simulink model "s8_15"  (Simulink 6.6)
settings: Solver=ode23  SolverMode=SingleTasking  StartTime=0.0  StopTime=t_d  MaxStep=Tc  RelTol=1e-8  AbsTol=1e-8
values from neighbouring files (symbols this model uses):
  F_v = K_r*diag([0.01 0.01])*K_r    [i8_15.m]
  g = 9.81    [i8_15.m]
  K_d = 3250*diag([1 1])    [i8_15.m]
  K_p = 16250*diag([1 1])    [i8_15.m]
  p_d = [0.6; -0.2]    [i8_15.m]
  pi_m = pi_l    [i8_15.m]
  q_i = inv_k2u(a,p_i)    [i8_15.m]
  Tc = 0.001    [i8_15.m]
  Ts = Tc    (= 0.001)    [i8_15.m]
undefined symbols (not defined in the file or in its folder): a, iner_l, pi_l
settings Model: Creator=luigivillani  LastModifiedBy=luigivillani  ExtModeAutoUpdateStatusClock=off
settings SolverCC: InitialStep=0.1*Tc
settings DataIOCC: LimitDataPoints=off  SaveOutput=off  SaveTime=off
settings OptimizationCC: BlockReduction=off  BooleanDataType=off
settings DebuggingCC: SignalResolutionControl=TryResolveAllWithWarning  SolverPrmCheckMsg=none  MultiTaskDSMMsg=warning  MultiTaskCondExecSysMsg=none  StrictBusMsg=None
settings HardwareCC: TargetUnknown=on
settings RTWCC: IncludeERTFirstTime=on

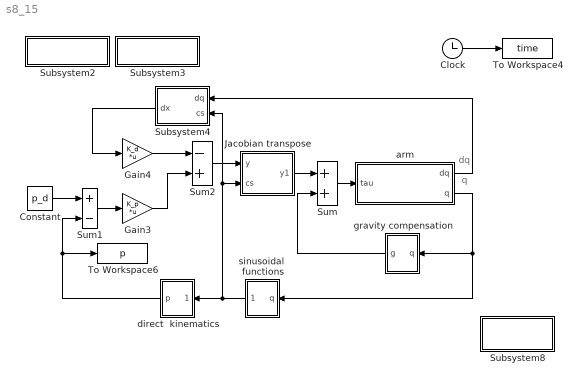
== system s8_15 ==
  note: dq
  note: q
  Clock : Clock
  Constant : Constant  Value=p_d
  Gain3 : Gain  Gain=K_p  Multiplication=Matrix(K*u)  SampleTime=Tc
      mask Display: disp('K_p')
  Gain4 : Gain  Gain=K_d  Multiplication=Matrix(K*u)  SampleTime=Tc
      mask Display: disp('K_d')
  Jacobian transpose : Subsystem
      mask Display: disp('tr(J_a(q))')
  Subsystem2 : Subsystem
      settings: OpenFcn=clear all;c=0;i8_15;
      mask Display: disp('p_d=[0.5 0.5]')
  Subsystem3 : Subsystem
      settings: OpenFcn=clear all;c=1;i8_15;
      mask Display: disp('p_d=[0.6 -0.2]')
  Subsystem4 : Subsystem  Orientation=left
      mask Display: disp('J_a(q)')
  Subsystem8 : Subsystem  Orientation=left
      settings: OpenFcn=p8_15;
      mask Display: disp('plot')
  Sum : Sum  SaturateOnIntegerOverflow=on  InputSameDT=on
  Sum1 : Sum  Inputs=+-  SaturateOnIntegerOverflow=on  InputSameDT=on
  Sum2 : Sum  Inputs=-+  SaturateOnIntegerOverflow=on  InputSameDT=on
  To Workspace4 : ToWorkspace  VariableName=time  SampleTime=Ts  SaveFormat=Array
      settings: MaxDataPoints=4001
  To Workspace6 : ToWorkspace  VariableName=p  SampleTime=Ts  SaveFormat=Array
      settings: MaxDataPoints=4001
  arm : Subsystem
      mask Display: disp('inv(B(q))(tau-tau'')')
  direct  kinematics : Subsystem  Orientation=left
      mask Display: disp('k(q)')
  gravity compensation : Subsystem  Orientation=left
      mask Display: disp('g(q)')
  sinusoidal  functions : Subsystem  Orientation=left
      mask Display: disp('cs(q)')
  wires:
  Sum/1 -> arm/1(tau)
  Sum1/1 -> Gain3/1
  Clock/1 -> To Workspace4/1
  Constant/1 -> Sum1/1
  gravity compensation/1(g) -> Sum/2
  Jacobian transpose/1(y1) -> Sum/1
  arm/2("q ") -> gravity compensation/1(q), sinusoidal  functions/1(q)
  Sum2/1 -> Jacobian transpose/1(y)
  Gain4/1 -> Sum2/1
  Subsystem4/1(dx) -> Gain4/1
  Gain3/1 -> Sum2/2
  arm/1(dq) -> Subsystem4/1(dq)
  sinusoidal  functions/1(cs) -> Subsystem4/2(cs), Jacobian transpose/2(cs), direct  kinematics/1(cs)
  direct  kinematics/1(p) -> Sum1/2, To Workspace6/1

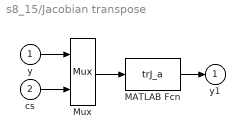
== system s8_15/Jacobian transpose ==
  y : Inport
  cs : Inport  Port=2
  MATLAB Fcn : MATLABFcn  MATLABFcn=trJ_a  OutputDimensions=2  SampleTime=Tc
      mask Display: disp('J''_a(q)y')
  Mux : Mux  Inputs=[2,4]
  y1 : Outport  InitialOutput=0
  wires:
  MATLAB Fcn/1 -> y1/1
  Mux/1 -> MATLAB Fcn/1
  cs/1 -> Mux/2
  y/1 -> Mux/1

== system s8_15/Subsystem2 ==
  note: start

== system s8_15/Subsystem3 ==
  note: start

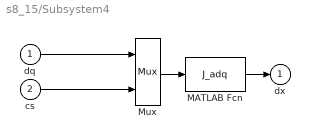
== system s8_15/Subsystem4 ==
  dq : Inport
  cs : Inport  Port=2
  MATLAB Fcn : MATLABFcn  MATLABFcn=J_adq  OutputDimensions=2  SampleTime=Tc
      mask Display: disp('J_a(q)dq')
  Mux : Mux  Inputs=[2,4]
  dx : Outport  InitialOutput=0
  wires:
  dq/1 -> Mux/1
  cs/1 -> Mux/2
  Mux/1 -> MATLAB Fcn/1
  MATLAB Fcn/1 -> dx/1

== system s8_15/Subsystem8 ==
  note: start

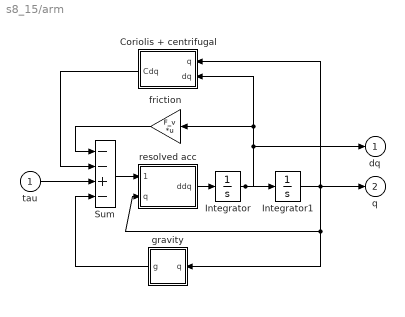
== system s8_15/arm ==
  tau : Inport
  Coriolis + centrifugal : Subsystem  Orientation=left
      mask Display: disp('C(q,dq)dq')
  Integrator : Integrator  InitialCondition=[0 0]  ZeroCross=off
  Integrator1 : Integrator  InitialCondition=q_i  ZeroCross=off
  Sum : Sum  Inputs=--+-  SaturateOnIntegerOverflow=on  InputSameDT=on
  friction : Gain  Orientation=left  Gain=F_v  Multiplication=Matrix(K*u)  SaturateOnIntegerOverflow=on
      mask Display: disp('F_v')
  gravity : Subsystem  Orientation=left
      mask Display: disp('g(q)')
  resolved acc : Subsystem
      mask Display: disp('inv(B(q))')
  dq : Outport  InitialOutput=0
  "q " : Outport  Port=2  InitialOutput=0
  wires:
  Coriolis + centrifugal/1(Cdq) -> Sum/2
  tau/1 -> Sum/3
  Integrator1/1 -> Coriolis + centrifugal/1(q), resolved acc/2(q), gravity/1(q), "q "/1
  resolved acc/1(ddq) -> Integrator/1
  Integrator/1 -> Integrator1/1, dq/1, Coriolis + centrifugal/2(dq), friction/1
  Sum/1 -> resolved acc/1(tau-tau')
  friction/1 -> Sum/1
  gravity/1(g) -> Sum/4

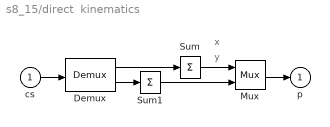
== system s8_15/direct  kinematics ==
  note: y
  note: x
  cs : Inport
  Demux : Demux  Outputs=[2,2]
  Mux : Mux  Inputs=2
  Sum : Sum  Inputs=+  SaturateOnIntegerOverflow=on  InputSameDT=on
  Sum1 : Sum  Inputs=+  SaturateOnIntegerOverflow=on  InputSameDT=on
  p : Outport  InitialOutput=0
  wires:
  Sum1/1 -> Mux/2
  Sum/1 -> Mux/1
  Demux/2 -> Sum1/1
  Demux/1 -> Sum/1
  cs/1 -> Demux/1
  Mux/1 -> p/1

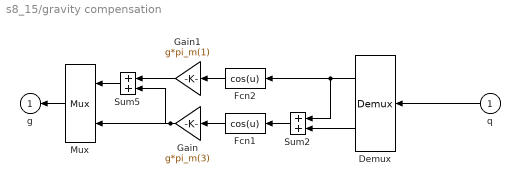
== system s8_15/gravity compensation ==
  q : Inport  Orientation=left
  Demux : Demux  Orientation=left  Outputs=2
  Fcn1 : Fcn  Orientation=left  Expr=cos(u)  SampleTime=Tc
  Fcn2 : Fcn  Orientation=left  Expr=cos(u)  SampleTime=Tc
  Gain : Gain  Orientation=left  Gain=g*pi_m(3)  SaturateOnIntegerOverflow=on
      mask Display: disp('k_2')
  Gain1 : Gain  Orientation=left  Gain=g*pi_m(1)  SaturateOnIntegerOverflow=on
      mask Display: disp('k_1')
  Mux : Mux  Orientation=left  Inputs=2
  Sum2 : Sum  Orientation=left  SampleTime=Tc  SaturateOnIntegerOverflow=on  InputSameDT=on
  Sum5 : Sum  Orientation=left  SaturateOnIntegerOverflow=on  InputSameDT=on
  g : Outport  Orientation=left  InitialOutput=0
  wires:
  Mux/1 -> g/1
  Gain/1 -> Sum5/2, Mux/2
  Sum5/1 -> Mux/1
  Gain1/1 -> Sum5/1
  Demux/1 -> Fcn2/1, Sum2/1
  Fcn2/1 -> Gain1/1
  Fcn1/1 -> Gain/1
  Sum2/1 -> Fcn1/1
  Demux/2 -> Sum2/2
  q/1 -> Demux/1

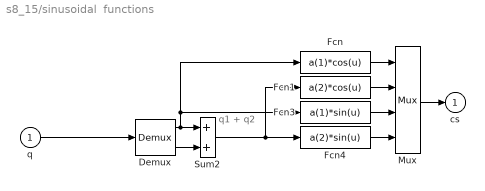
== system s8_15/sinusoidal  functions ==
  note: q1 + q2
  q : Inport
  Demux : Demux  Outputs=2
  Fcn : Fcn  Expr=a(1)*cos(u)  SampleTime=Tc
  Fcn1 : Fcn  Expr=a(2)*cos(u)  SampleTime=Tc
  Fcn3 : Fcn  Expr=a(1)*sin(u)  SampleTime=Tc
  Fcn4 : Fcn  Expr=a(2)*sin(u)  SampleTime=Tc
  Mux : Mux
  Sum2 : Sum  SampleTime=Tc  SaturateOnIntegerOverflow=on  InputSameDT=on
  cs : Outport  InitialOutput=0
  wires:
  Fcn/1 -> Mux/1
  Mux/1 -> cs/1
  Demux/2 -> Sum2/2
  Sum2/1 -> Fcn1/1, Fcn4/1
  Demux/1 -> Sum2/1, Fcn/1, Fcn3/1
  Fcn1/1 -> Mux/2
  Fcn3/1 -> Mux/3
  Fcn4/1 -> Mux/4
  q/1 -> Demux/1

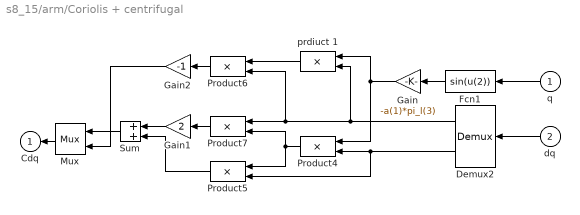
== system s8_15/arm/Coriolis + centrifugal ==
  q : Inport  Orientation=left
  dq : Inport  Orientation=left  Port=2
  Demux2 : Demux  Orientation=left  Outputs=2
  Fcn1 : Fcn  Orientation=left  Expr=sin(u(2))
  Gain : Gain  Orientation=left  Gain=-a(1)*pi_l(3)  SaturateOnIntegerOverflow=on
      mask Display: disp('k_3')
  Gain1 : Gain  Orientation=left  Gain=2  SaturateOnIntegerOverflow=on
  Gain2 : Gain  Orientation=left  Gain=-1  SaturateOnIntegerOverflow=on
  Mux : Mux  Orientation=left  Inputs=2
  Product{4..7} (4 alike) : Product  Orientation=left  SaturateOnIntegerOverflow=on  RndMeth=Zero  InputSameDT=on
  Sum : Sum  Orientation=left  SaturateOnIntegerOverflow=on  InputSameDT=on
  prdiuct 1 : Product  Orientation=left  SaturateOnIntegerOverflow=on  RndMeth=Zero  InputSameDT=on
  Cdq : Outport  Orientation=left  InitialOutput=0
  wires:
  dq/1 -> Demux2/1
  Gain2/1 -> Mux/2
  Product6/1 -> Gain2/1
  Mux/1 -> Cdq/1
  Sum/1 -> Mux/1
  Product5/1 -> Sum/2
  Gain1/1 -> Sum/1
  Product7/1 -> Gain1/1
  Demux2/1 -> prdiuct 1/2, Product6/2, Product7/1
  Demux2/2 -> Product4/2, Product5/2
  prdiuct 1/1 -> Product6/1
  Gain/1 -> prdiuct 1/1, Product4/1
  Fcn1/1 -> Gain/1
  q/1 -> Fcn1/1
  Product4/1 -> Product5/1, Product7/2

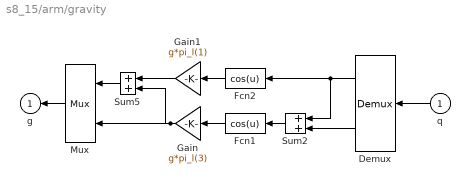
== system s8_15/arm/gravity ==
  q : Inport  Orientation=left
  Demux : Demux  Orientation=left  Outputs=2
  Fcn1 : Fcn  Orientation=left  Expr=cos(u)
  Fcn2 : Fcn  Orientation=left  Expr=cos(u)
  Gain : Gain  Orientation=left  Gain=g*pi_l(3)  SaturateOnIntegerOverflow=on
      mask Display: disp('k_2')
  Gain1 : Gain  Orientation=left  Gain=g*pi_l(1)  SaturateOnIntegerOverflow=on
      mask Display: disp('k_1')
  Mux : Mux  Orientation=left  Inputs=2
  Sum2 : Sum  Orientation=left  SaturateOnIntegerOverflow=on  InputSameDT=on
  Sum5 : Sum  Orientation=left  SaturateOnIntegerOverflow=on  InputSameDT=on
  g : Outport  Orientation=left  InitialOutput=0
  wires:
  q/1 -> Demux/1
  Demux/2 -> Sum2/2
  Sum2/1 -> Fcn1/1
  Fcn1/1 -> Gain/1
  Fcn2/1 -> Gain1/1
  Demux/1 -> Fcn2/1, Sum2/1
  Gain1/1 -> Sum5/1
  Sum5/1 -> Mux/1
  Gain/1 -> Sum5/2, Mux/2
  Mux/1 -> g/1

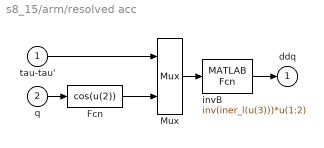
== system s8_15/arm/resolved acc ==
  tau-tau' : Inport
  q : Inport  Port=2
  Fcn : Fcn  Expr=cos(u(2))
  Mux : Mux  Inputs=[2,1]
  "invB " : MATLABFcn  MATLABFcn=inv(iner_l(u(3)))*u(1:2)  OutputDimensions=2
      mask Display: disp('inv(B(q))')
  ddq : Outport  InitialOutput=0
  wires:
  Fcn/1 -> Mux/2
  q/1 -> Fcn/1
  "invB "/1 -> ddq/1
  tau-tau'/1 -> Mux/1
  Mux/1 -> "invB "/1
